simulink library "Brakes_Pedal"  (R2020a)
settings: Solver=VariableStepAuto  StartTime=0.0  StopTime=10.0  RelTol=1e-3
undefined symbols (not defined in the file): Brakes
libraries: nesl_utility x12, sdl_lib x6, fl_lib x6
Description:
  | Component of Simscape Vehicle Templates Library
  | 
  | Copyright 2018-2020 The MathWorks, Inc.
settings Model: Creator=smiller  LastModifiedBy=smiller
settings DataIOCC: ReturnWorkspaceOutputs=off
settings DebuggingCC: ArithmeticOperatorsInVariantConditions=warning
settings SFSimCC: CustomCodeUndefinedFunction=UseInterfaceOnly

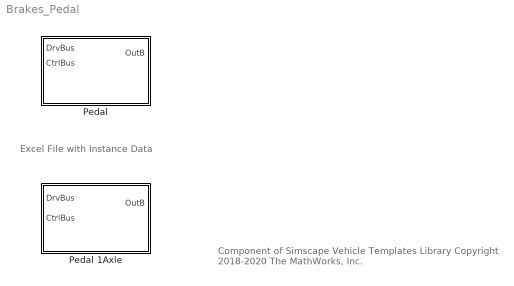
== system Brakes_Pedal ==
  note: Excel File with Instance Data
  note: Component of Simscape Vehicle Templates Library
      | Copyright 2018-2020 The MathWorks, Inc.
  Pedal : Subsystem  Tag=PublishSubsystem  VariantControl=Pedal  mask(Brake System, Pedal Input){brk_pad_rad_fa=Brakes.Front.DiscAndPad.lMeanRadius.Value, brk_pad_rad_ra=Brakes.Rear.DiscAndPad.lMeanRadius.Value, brk_cyl_bore_fa=Brakes.Front.Caliper.lCylinderDiameter.Value, brk_cyl_bore_ra=Brakes.Rear.Caliper.lCylinderDiameter.Value, brk_n_pads_fa=Brakes.Front.DiscAndPad.NPads.Value, brk_n_pads_ra=Brakes.Rear.DiscAndPad.NPads.Value, brk_mu_static_fa=Brakes.Front.DiscAndPad.rMuStatic.Value, brk_mu_static_ra=Brakes.Rear.DiscAndPad.rMuStatic.Value, brk_mu_kin_fa=Brakes.Front.DiscAndPad.rMuKinetic.Value, brk_mu_kin_ra=Brakes.Rear.DiscAndPad.rMuKinetic.Value, brk_trans_vel_fa=Brakes.Front.DiscAndPad.nTransition.Value, brk_trans_vel_ra=Brakes.Rear.DiscAndPad.nTransition.Value, brk_visc_coef_fa=Brakes.Front.DiscAndPad.dViscous.Value, brk_visc_coef_ra=Brakes.Rear.DiscAndPad.dViscous.Value, brk_max_p_fa=Brakes.Front.Caliper.pMax.Value, brk_max_p_ra=Brakes.Rear.Caliper.pMax.Value, brk_filt_fa=1/Brakes.Front.Caliper.fActuatorCutoff.Value, brk_filt_ra=1/Brakes.Rear.Caliper.fActuatorCutoff.Value}
      mask TypeOptions brk_pad_rad_fa:
      | Disc
      | Brake
      | FL/r_mean | Disc
      | Brake
      | FR/r_mean
      mask TypeOptions brk_pad_rad_ra:
      | Disc
      | Brake
      | RL/r_mean | Disc
      | Brake
      | RR/r_mean
      mask TypeOptions brk_cyl_bore_fa:
      | Disc
      | Brake
      | FL/bore | Disc
      | Brake
      | FR/bore
      mask TypeOptions brk_cyl_bore_ra:
      | Disc
      | Brake
      | RL/bore | Disc
      | Brake
      | RR/bore
      mask TypeOptions brk_n_pads_fa:
      | Disc
      | Brake
      | FL/n_pads | Disc
      | Brake
      | FR/n_pads
      mask TypeOptions brk_n_pads_ra:
      | Disc
      | Brake
      | RL/n_pads | Disc
      | Brake
      | RR/n_pads
      mask TypeOptions brk_mu_static_fa:
      | Disc
      | Brake
      | FL/mu_static | Disc
      | Brake
      | FR/mu_static
      mask TypeOptions brk_mu_static_ra:
      | Disc
      | Brake
      | RL/mu_static | Disc
      | Brake
      | RR/mu_static
      mask TypeOptions brk_mu_kin_fa:
      | Disc
      | Brake
      | FL/mu_coulomb | Disc
      | Brake
      | FR/mu_coulomb
      mask TypeOptions brk_mu_kin_ra:
      | Disc
      | Brake
      | RL/mu_coulomb | Disc
      | Brake
      | RR/mu_coulomb
      mask TypeOptions brk_trans_vel_fa:
      | Disc
      | Brake
      | FL/brkwy_vel | Disc
      | Brake
      | FR/brkwy_vel
      mask TypeOptions brk_trans_vel_ra:
      | Disc
      | Brake
      | RL/brkwy_vel | Disc
      | Brake
      | RR/brkwy_vel
      mask TypeOptions brk_visc_coef_fa:
      | Disc
      | Brake
      | FL/visc_coef | Disc
      | Brake
      | FR/visc_coef
      mask TypeOptions brk_visc_coef_ra:
      | Disc
      | Brake
      | RL/visc_coef | Disc
      | Brake
      | RR/visc_coef
      mask TypeOptions brk_max_p_fa: Actuator FL/brk_max_p | Actuator FR/brk_max_p
      mask TypeOptions brk_max_p_ra: Actuator RL/brk_max_p | Actuator RR/brk_max_p
      mask TypeOptions brk_filt_fa: Actuator FL/brk_filt | Actuator FR/brk_filt
      mask TypeOptions brk_filt_ra: Actuator RL/brk_filt | Actuator RR/brk_filt
      mask DialogControl cont_brakes Prompt: Brakes
      mask DialogControl cont_brk_geom Prompt: Geometry
      mask DialogControl text_brakes_fa Prompt: Front Susp.
      mask DialogControl text_brakes_ra Prompt: Rear Susp.
      mask DialogControl text_brakes_pad_rad Prompt: Mean Pad Radius (m)
      mask DialogControl text_brakes_cyl_bore Prompt: Cylinder Bore (m)
      mask DialogControl text_brakes_n_pads Prompt: Number of pads
      mask DialogControl cont_brk_frict Prompt: Friction
      mask DialogControl text_brakes_mu_static Prompt: Static Coeff. (0-1)
      mask DialogControl text_brakes_mu_kin Prompt: Kinetic Coeff. (0-1)
      mask DialogControl text_brakes_trans_vel Prompt: Trans. Velocity (rad/s)
      mask DialogControl text_brakes_visc_coef Prompt: Viscous (N*m/(rad/s))
      mask DialogControl cont_brk_act Prompt: Actuator
      mask DialogControl text_brakes_maxp Prompt: Max Pad Pressure (Pa)
      mask DialogControl text_brakes_filt Prompt: Time Constant (s)
      mask Display: image('sm_car_vehicle_brakes_pedal_IMAGE.png');
  Pedal 1Axle : Subsystem  Tag=PublishSubsystem  VariantControl=Pedal  mask(Brake System, Pedal Input){brk_pad_rad_fa=Brakes.Front.DiscAndPad.lMeanRadius.Value, brk_cyl_bore_fa=Brakes.Front.Caliper.lCylinderDiameter.Value, brk_n_pads_fa=Brakes.Front.DiscAndPad.NPads.Value, brk_mu_static_fa=Brakes.Front.DiscAndPad.rMuStatic.Value, brk_mu_kin_fa=Brakes.Front.DiscAndPad.rMuKinetic.Value, brk_trans_vel_fa=Brakes.Front.DiscAndPad.nTransition.Value, brk_visc_coef_fa=Brakes.Front.DiscAndPad.dViscous.Value, brk_max_p_fa=Brakes.Front.Caliper.pMax.Value, brk_filt_fa=1/Brakes.Front.Caliper.fActuatorCutoff.Value}
      mask TypeOptions brk_pad_rad_fa:
      | Disc
      | Brake
      | FL/r_mean | Disc
      | Brake
      | FR/r_mean
      mask TypeOptions brk_cyl_bore_fa:
      | Disc
      | Brake
      | FL/bore | Disc
      | Brake
      | FR/bore
      mask TypeOptions brk_n_pads_fa:
      | Disc
      | Brake
      | FL/n_pads | Disc
      | Brake
      | FR/n_pads
      mask TypeOptions brk_mu_static_fa:
      | Disc
      | Brake
      | FL/mu_static | Disc
      | Brake
      | FR/mu_static
      mask TypeOptions brk_mu_kin_fa:
      | Disc
      | Brake
      | FL/mu_coulomb | Disc
      | Brake
      | FR/mu_coulomb
      mask TypeOptions brk_trans_vel_fa:
      | Disc
      | Brake
      | FL/brkwy_vel | Disc
      | Brake
      | FR/brkwy_vel
      mask TypeOptions brk_visc_coef_fa:
      | Disc
      | Brake
      | FL/visc_coef | Disc
      | Brake
      | FR/visc_coef
      mask TypeOptions brk_max_p_fa: Actuator FL/brk_max_p | Actuator FR/brk_max_p
      mask TypeOptions brk_filt_fa: Actuator FL/brk_filt | Actuator FR/brk_filt
      mask DialogControl cont_brakes Prompt: Brakes
      mask DialogControl cont_brk_geom Prompt: Geometry
      mask DialogControl text_brakes_fa Prompt: Front Susp.
      mask DialogControl text_brakes_pad_rad Prompt: Mean Pad Radius (m)
      mask DialogControl text_brakes_cyl_bore Prompt: Cylinder Bore (m)
      mask DialogControl text_brakes_n_pads Prompt: Number of pads
      mask DialogControl cont_brk_frict Prompt: Friction
      mask DialogControl text_brakes_mu_static Prompt: Static Coeff. (0-1)
      mask DialogControl text_brakes_mu_kin Prompt: Kinetic Coeff. (0-1)
      mask DialogControl text_brakes_trans_vel Prompt: Trans. Velocity (rad/s)
      mask DialogControl text_brakes_visc_coef Prompt: Viscous (N*m/(rad/s))
      mask DialogControl cont_brk_act Prompt: Actuator
      mask DialogControl text_brakes_maxp Prompt: Max Pad Pressure (Pa)
      mask DialogControl text_brakes_filt Prompt: Time Constant (s)
      mask Display: image('sm_car_vehicle_brakes_pedal_IMAGE.png');

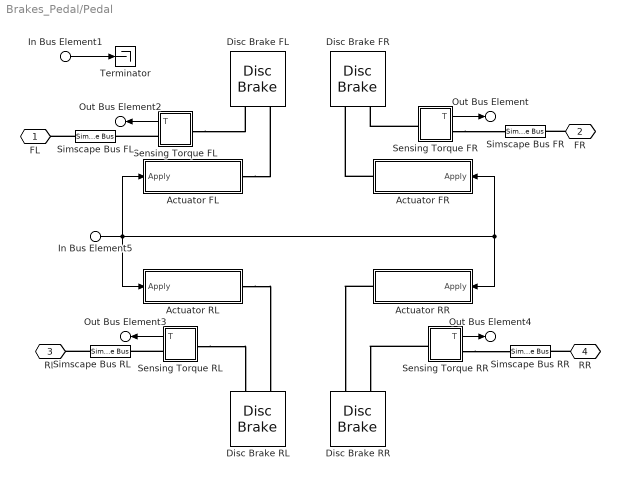
== system Brakes_Pedal/Pedal ==
  In Bus Element5 : Inport  PortName=DrvBus  Element=rBrakePedal
  In Bus Element1 : Inport  Port=2  PortName=CtrlBus
  Actuator FL : Subsystem  mask{brk_max_p=brk_max_p_fa, brk_filt=brk_filt_fa}
      mask prompts: brk_max_p "Max Pad Pressure (Pa)"; brk_filt "Time Constant (s)"
      mask TypeOptions brk_max_p: Filter/Numerator
  Actuator FR : Subsystem  mask{brk_max_p=brk_max_p_fa, brk_filt=brk_filt_fa}
      mask prompts: brk_max_p "Max Pad Pressure (Pa)"; brk_filt "Time Constant (s)"
      mask TypeOptions brk_max_p: Filter/Numerator
  Actuator RL : Subsystem  mask{brk_max_p=brk_max_p_ra, brk_filt=brk_filt_ra}
      mask prompts: brk_max_p "Max Pad Pressure (Pa)"; brk_filt "Time Constant (s)"
      mask TypeOptions brk_max_p: Filter/Numerator
  Actuator RR : Subsystem  mask{brk_max_p=brk_max_p_ra, brk_filt=brk_filt_ra}
      mask prompts: brk_max_p "Max Pad Pressure (Pa)"; brk_filt "Time Constant (s)"
      mask TypeOptions brk_max_p: Filter/Numerator
  Disc Brake FL : sdl_lib/Brakes & Detents/Rotational/Disc Brake  r_mean=brk_pad_rad_fa m  bore=brk_cyl_bore_fa m  n_pads=brk_n_pads_fa  thermal_port=simscape.enum.thermaleffects.omit  mu_static=brk_mu_static_fa  mu_coulomb=brk_mu_kin_fa  temperature_TLU=[280, 300, 320] K  mu_static_TLU=[.9, .8, .7]  mu_coulomb_TLU=[.8, .7, .6]  thermal_mass=50 kJ/K  brkwy_vel=brk_trans_vel_fa rad/s  visc_coef=brk_visc_coef_fa N*m/(rad/s)  temperature_specify=off  temperature_priority=High  temperature=300 K  temperature_nominal_specify=off  temperature_nominal_unit=K  temperature_nominal_value=1
      settings: SourceProductBaseCode=LD
  Disc Brake FR : sdl_lib/Brakes & Detents/Rotational/Disc Brake  r_mean=brk_pad_rad_fa m  bore=brk_cyl_bore_fa m  n_pads=brk_n_pads_fa  thermal_port=simscape.enum.thermaleffects.omit  mu_static=brk_mu_static_fa  mu_coulomb=brk_mu_kin_fa  temperature_TLU=[280, 300, 320] K  mu_static_TLU=[.9, .8, .7]  mu_coulomb_TLU=[.8, .7, .6]  thermal_mass=50 kJ/K  brkwy_vel=brk_trans_vel_fa rad/s  visc_coef=brk_visc_coef_fa N*m/(rad/s)  temperature_specify=off  temperature_priority=High  temperature=300 K  temperature_nominal_specify=off  temperature_nominal_unit=K  temperature_nominal_value=1
      settings: SourceProductBaseCode=LD
  Disc Brake RL : sdl_lib/Brakes & Detents/Rotational/Disc Brake  r_mean=brk_pad_rad_ra m  bore=brk_cyl_bore_ra m  n_pads=brk_n_pads_ra  thermal_port=simscape.enum.thermaleffects.omit  mu_static=brk_mu_static_ra  mu_coulomb=brk_mu_kin_ra  temperature_TLU=[280, 300, 320] K  mu_static_TLU=[.9, .8, .7]  mu_coulomb_TLU=[.8, .7, .6]  thermal_mass=50 kJ/K  brkwy_vel=brk_trans_vel_ra rad/s  visc_coef=brk_visc_coef_ra N*m/(rad/s)  temperature_specify=off  temperature_priority=High  temperature=300 K  temperature_nominal_specify=off  temperature_nominal_unit=K  temperature_nominal_value=1
      settings: SourceProductBaseCode=LD
  Disc Brake RR : sdl_lib/Brakes & Detents/Rotational/Disc Brake  r_mean=brk_pad_rad_ra m  bore=brk_cyl_bore_ra m  n_pads=brk_n_pads_ra  thermal_port=simscape.enum.thermaleffects.omit  mu_static=brk_mu_static_ra  mu_coulomb=brk_mu_kin_ra  temperature_TLU=[280, 300, 320] K  mu_static_TLU=[.9, .8, .7]  mu_coulomb_TLU=[.8, .7, .6]  thermal_mass=50 kJ/K  brkwy_vel=brk_trans_vel_ra rad/s  visc_coef=brk_visc_coef_ra N*m/(rad/s)  temperature_specify=off  temperature_priority=High  temperature=300 K  temperature_nominal_specify=off  temperature_nominal_unit=K  temperature_nominal_value=1
      settings: SourceProductBaseCode=LD
  Sensing Torque FL : Subsystem
  Sensing Torque FR : Subsystem
  Sensing Torque RL : Subsystem
  Sensing Torque RR : Subsystem
  Simscape Bus FL : SimscapeBus  HierarchyStrings=Axle1D
  Simscape Bus FR : SimscapeBus  HierarchyStrings=Axle1D
  Simscape Bus RL : SimscapeBus  HierarchyStrings=Axle1D
  Simscape Bus RR : SimscapeBus  HierarchyStrings=Axle1D
  Terminator : Terminator
  FL : PMIOPort  Side=Left
  FR : PMIOPort  Port=2  Side=Right
  RL : PMIOPort  Port=3  Side=Left
  RR : PMIOPort  Port=4  Side=Right
  Out Bus Element2 : Outport  VectorParamsAs1DForOutWhenUnconnected=off  PortName=OutB  Element=MBrakeFL
  Out Bus Element : Outport  VectorParamsAs1DForOutWhenUnconnected=off  PortName=OutB  Element=MBrakeFR
  Out Bus Element3 : Outport  VectorParamsAs1DForOutWhenUnconnected=off  PortName=OutB  Element=MBrakeRL
  Out Bus Element4 : Outport  VectorParamsAs1DForOutWhenUnconnected=off  PortName=OutB  Element=MBrakeRR
  wires:
  Sensing Torque RR/1(T) -> Out Bus Element4/1
  Sensing Torque RL/1(T) -> Out Bus Element3/1
  Sensing Torque FR/1(T) -> Out Bus Element/1
  Sensing Torque FL/1(T) -> Out Bus Element2/1
  In Bus Element1/1 -> Terminator/1
  In Bus Element5/1 -> Actuator RR/1(Apply), Actuator FR/1(Apply), Actuator FL/1(Apply), Actuator RL/1(Apply)
  connections:
  Sensing Torque RR/RConn1 -- Simscape Bus RR/LConn1
  Sensing Torque RL/RConn1 -- Simscape Bus RL/LConn1
  Sensing Torque FR/RConn1 -- Simscape Bus FR/LConn1
  Sensing Torque FL/RConn1 -- Simscape Bus FL/LConn1
  Sensing Torque FL/LConn1 -- Disc Brake FL/LConn2
  Simscape Bus FL/RConn1 -- FL/RConn1
  Sensing Torque RL/LConn1 -- Disc Brake RL/LConn2
  Simscape Bus RL/RConn1 -- RL/RConn1
  RR/RConn1 -- Simscape Bus RR/RConn1
  FR/RConn1 -- Simscape Bus FR/RConn1
  Actuator RR/RConn1 -- Disc Brake RR/LConn1
  Actuator FL/RConn1 -- Disc Brake FL/LConn1
  Actuator RL/RConn1 -- Disc Brake RL/LConn1
  Actuator FR/RConn1 -- Disc Brake FR/LConn1
  Sensing Torque FR/LConn1 -- Disc Brake FR/LConn2
  Sensing Torque RR/LConn1 -- Disc Brake RR/LConn2

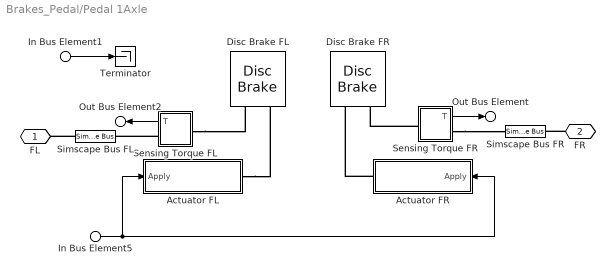
== system Brakes_Pedal/Pedal 1Axle ==
  In Bus Element5 : Inport  PortName=DrvBus  Element=rBrakePedal
  In Bus Element1 : Inport  Port=2  PortName=CtrlBus
  Actuator FL : Subsystem  mask{brk_max_p=brk_max_p_fa, brk_filt=brk_filt_fa}
      mask prompts: brk_max_p "Max Pad Pressure (Pa)"; brk_filt "Time Constant (s)"
      mask TypeOptions brk_max_p: Filter/Numerator
  Actuator FR : Subsystem  mask{brk_max_p=brk_max_p_fa, brk_filt=brk_filt_fa}
      mask prompts: brk_max_p "Max Pad Pressure (Pa)"; brk_filt "Time Constant (s)"
      mask TypeOptions brk_max_p: Filter/Numerator
  Disc Brake FL : sdl_lib/Brakes & Detents/Rotational/Disc Brake  r_mean=brk_pad_rad_fa m  bore=brk_cyl_bore_fa m  n_pads=brk_n_pads_fa  thermal_port=simscape.enum.thermaleffects.omit  mu_static=brk_mu_static_fa  mu_coulomb=brk_mu_kin_fa  temperature_TLU=[280, 300, 320] K  mu_static_TLU=[.9, .8, .7]  mu_coulomb_TLU=[.8, .7, .6]  thermal_mass=50 kJ/K  brkwy_vel=brk_trans_vel_fa rad/s  visc_coef=brk_visc_coef_fa N*m/(rad/s)  temperature_specify=off  temperature_priority=High  temperature=300 K  temperature_nominal_specify=off  temperature_nominal_unit=K  temperature_nominal_value=1
      settings: SourceProductBaseCode=LD
  Disc Brake FR : sdl_lib/Brakes & Detents/Rotational/Disc Brake  r_mean=brk_pad_rad_fa m  bore=brk_cyl_bore_fa m  n_pads=brk_n_pads_fa  thermal_port=simscape.enum.thermaleffects.omit  mu_static=brk_mu_static_fa  mu_coulomb=brk_mu_kin_fa  temperature_TLU=[280, 300, 320] K  mu_static_TLU=[.9, .8, .7]  mu_coulomb_TLU=[.8, .7, .6]  thermal_mass=50 kJ/K  brkwy_vel=brk_trans_vel_fa rad/s  visc_coef=brk_visc_coef_fa N*m/(rad/s)  temperature_specify=off  temperature_priority=High  temperature=300 K  temperature_nominal_specify=off  temperature_nominal_unit=K  temperature_nominal_value=1
      settings: SourceProductBaseCode=LD
  Sensing Torque FL : Subsystem
  Sensing Torque FR : Subsystem
  Simscape Bus FL : SimscapeBus  HierarchyStrings=Axle1D
  Simscape Bus FR : SimscapeBus  HierarchyStrings=Axle1D
  Terminator : Terminator
  FL : PMIOPort  Side=Left
  FR : PMIOPort  Port=2  Side=Right
  Out Bus Element2 : Outport  VectorParamsAs1DForOutWhenUnconnected=off  PortName=OutB  Element=MBrakeFL
  Out Bus Element : Outport  VectorParamsAs1DForOutWhenUnconnected=off  PortName=OutB  Element=MBrakeFR
  wires:
  In Bus Element5/1 -> Actuator FL/1(Apply), Actuator FR/1(Apply)
  In Bus Element1/1 -> Terminator/1
  Sensing Torque FL/1(T) -> Out Bus Element2/1
  Sensing Torque FR/1(T) -> Out Bus Element/1
  connections:
  Sensing Torque FR/LConn1 -- Disc Brake FR/LConn2
  Actuator FR/RConn1 -- Disc Brake FR/LConn1
  Actuator FL/RConn1 -- Disc Brake FL/LConn1
  FR/RConn1 -- Simscape Bus FR/RConn1
  Simscape Bus FL/RConn1 -- FL/RConn1
  Sensing Torque FL/LConn1 -- Disc Brake FL/LConn2
  Sensing Torque FL/RConn1 -- Simscape Bus FL/LConn1
  Sensing Torque FR/RConn1 -- Simscape Bus FR/LConn1

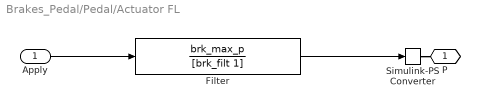
== system Brakes_Pedal/Pedal/Actuator FL ==
  Apply : Inport
  Filter : TransferFcn  Numerator=brk_max_p  Denominator=[brk_filt 1]
  Simulink-PS Converter : nesl_utility/Simulink-PS Converter  PhysicalDomain=network_engine_domain  SubClassName=ps_input  LeftPortType=input  RightPortType=output  PseudoPeriodic=off  Frequencies=[]  NoiseDistribution=none  NoiseParameters=[]  Unit=1  AffineConversion=off  FilteringAndDerivatives=provide  SimscapeFilterOrder=1  InputFilterTimeConstant=0.001  UdotUserProvided=0
  P : PMIOPort  Side=Right
  wires:
  Apply/1 -> Filter/1
  Filter/1 -> Simulink-PS Converter/1
  connections:
  Simulink-PS Converter/RConn1 -- P/RConn1

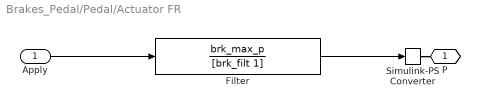
== system Brakes_Pedal/Pedal/Actuator FR ==
  Apply : Inport
  Filter : TransferFcn  Numerator=brk_max_p  Denominator=[brk_filt 1]
  Simulink-PS Converter : nesl_utility/Simulink-PS Converter  PhysicalDomain=network_engine_domain  SubClassName=ps_input  LeftPortType=input  RightPortType=output  PseudoPeriodic=off  Frequencies=[]  NoiseDistribution=none  NoiseParameters=[]  Unit=1  AffineConversion=off  FilteringAndDerivatives=provide  SimscapeFilterOrder=1  InputFilterTimeConstant=0.001  UdotUserProvided=0
  P : PMIOPort  Side=Right
  wires:
  Filter/1 -> Simulink-PS Converter/1
  Apply/1 -> Filter/1
  connections:
  Simulink-PS Converter/RConn1 -- P/RConn1

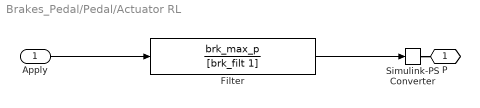
== system Brakes_Pedal/Pedal/Actuator RL ==
  Apply : Inport
  Filter : TransferFcn  Numerator=brk_max_p  Denominator=[brk_filt 1]
  Simulink-PS Converter : nesl_utility/Simulink-PS Converter  PhysicalDomain=network_engine_domain  SubClassName=ps_input  LeftPortType=input  RightPortType=output  PseudoPeriodic=off  Frequencies=[]  NoiseDistribution=none  NoiseParameters=[]  Unit=1  AffineConversion=off  FilteringAndDerivatives=provide  SimscapeFilterOrder=1  InputFilterTimeConstant=0.001  UdotUserProvided=0
  P : PMIOPort  Side=Right
  wires:
  Filter/1 -> Simulink-PS Converter/1
  Apply/1 -> Filter/1
  connections:
  Simulink-PS Converter/RConn1 -- P/RConn1

== system Brakes_Pedal/Pedal/Actuator RR ==
  Apply : Inport
  Filter : TransferFcn  Numerator=brk_max_p  Denominator=[brk_filt 1]
  Simulink-PS Converter : nesl_utility/Simulink-PS Converter  PhysicalDomain=network_engine_domain  SubClassName=ps_input  LeftPortType=input  RightPortType=output  PseudoPeriodic=off  Frequencies=[]  NoiseDistribution=none  NoiseParameters=[]  Unit=1  AffineConversion=off  FilteringAndDerivatives=provide  SimscapeFilterOrder=1  InputFilterTimeConstant=0.001  UdotUserProvided=0
  P : PMIOPort  Side=Right
  wires:
  Apply/1 -> Filter/1
  Filter/1 -> Simulink-PS Converter/1
  connections:
  Simulink-PS Converter/RConn1 -- P/RConn1

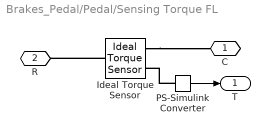
== system Brakes_Pedal/Pedal/Sensing Torque FL ==
  Ideal Torque Sensor : fl_lib/Mechanical/Mechanical Sensors/Ideal Torque Sensor
  PS-Simulink Converter : nesl_utility/PS-Simulink Converter  PhysicalDomain=network_engine_domain  SubClassName=ps_output  LeftPortType=input  RightPortType=output  PseudoPeriodic=off  Frequencies=[]  Unit=N*m  AffineConversion=off
  C : PMIOPort  Side=Right
  R : PMIOPort  Port=2  Side=Left
  T : Outport  VectorParamsAs1DForOutWhenUnconnected=off
  wires:
  PS-Simulink Converter/1 -> T/1
  connections:
  Ideal Torque Sensor/LConn1 -- R/RConn1
  Ideal Torque Sensor/RConn1 -- C/RConn1
  PS-Simulink Converter/LConn1 -- Ideal Torque Sensor/RConn2

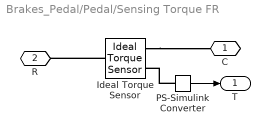
== system Brakes_Pedal/Pedal/Sensing Torque FR ==
  Ideal Torque Sensor : fl_lib/Mechanical/Mechanical Sensors/Ideal Torque Sensor
  PS-Simulink Converter : nesl_utility/PS-Simulink Converter  PhysicalDomain=network_engine_domain  SubClassName=ps_output  LeftPortType=input  RightPortType=output  PseudoPeriodic=off  Frequencies=[]  Unit=N*m  AffineConversion=off
  C : PMIOPort  Side=Right
  R : PMIOPort  Port=2  Side=Left
  T : Outport  VectorParamsAs1DForOutWhenUnconnected=off
  wires:
  PS-Simulink Converter/1 -> T/1
  connections:
  PS-Simulink Converter/LConn1 -- Ideal Torque Sensor/RConn2
  Ideal Torque Sensor/RConn1 -- C/RConn1
  Ideal Torque Sensor/LConn1 -- R/RConn1

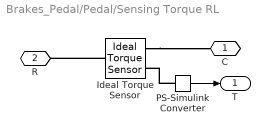
== system Brakes_Pedal/Pedal/Sensing Torque RL ==
  Ideal Torque Sensor : fl_lib/Mechanical/Mechanical Sensors/Ideal Torque Sensor
  PS-Simulink Converter : nesl_utility/PS-Simulink Converter  PhysicalDomain=network_engine_domain  SubClassName=ps_output  LeftPortType=input  RightPortType=output  PseudoPeriodic=off  Frequencies=[]  Unit=N*m  AffineConversion=off
  C : PMIOPort  Side=Right
  R : PMIOPort  Port=2  Side=Left
  T : Outport  VectorParamsAs1DForOutWhenUnconnected=off
  wires:
  PS-Simulink Converter/1 -> T/1
  connections:
  Ideal Torque Sensor/LConn1 -- R/RConn1
  Ideal Torque Sensor/RConn1 -- C/RConn1
  PS-Simulink Converter/LConn1 -- Ideal Torque Sensor/RConn2

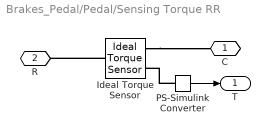
== system Brakes_Pedal/Pedal/Sensing Torque RR ==
  Ideal Torque Sensor : fl_lib/Mechanical/Mechanical Sensors/Ideal Torque Sensor
  PS-Simulink Converter : nesl_utility/PS-Simulink Converter  PhysicalDomain=network_engine_domain  SubClassName=ps_output  LeftPortType=input  RightPortType=output  PseudoPeriodic=off  Frequencies=[]  Unit=N*m  AffineConversion=off
  C : PMIOPort  Side=Right
  R : PMIOPort  Port=2  Side=Left
  T : Outport  VectorParamsAs1DForOutWhenUnconnected=off
  wires:
  PS-Simulink Converter/1 -> T/1
  connections:
  PS-Simulink Converter/LConn1 -- Ideal Torque Sensor/RConn2
  Ideal Torque Sensor/RConn1 -- C/RConn1
  Ideal Torque Sensor/LConn1 -- R/RConn1

== system Brakes_Pedal/Pedal 1Axle/Actuator FL ==
  Apply : Inport
  Filter : TransferFcn  Numerator=brk_max_p  Denominator=[brk_filt 1]
  Simulink-PS Converter : nesl_utility/Simulink-PS Converter  PhysicalDomain=network_engine_domain  SubClassName=ps_input  LeftPortType=input  RightPortType=output  PseudoPeriodic=off  Frequencies=[]  NoiseDistribution=none  NoiseParameters=[]  Unit=1  AffineConversion=off  FilteringAndDerivatives=provide  SimscapeFilterOrder=1  InputFilterTimeConstant=0.001  UdotUserProvided=0
  P : PMIOPort  Side=Right
  wires:
  Filter/1 -> Simulink-PS Converter/1
  Apply/1 -> Filter/1
  connections:
  Simulink-PS Converter/RConn1 -- P/RConn1

== system Brakes_Pedal/Pedal 1Axle/Actuator FR ==
  Apply : Inport
  Filter : TransferFcn  Numerator=brk_max_p  Denominator=[brk_filt 1]
  Simulink-PS Converter : nesl_utility/Simulink-PS Converter  PhysicalDomain=network_engine_domain  SubClassName=ps_input  LeftPortType=input  RightPortType=output  PseudoPeriodic=off  Frequencies=[]  NoiseDistribution=none  NoiseParameters=[]  Unit=1  AffineConversion=off  FilteringAndDerivatives=provide  SimscapeFilterOrder=1  InputFilterTimeConstant=0.001  UdotUserProvided=0
  P : PMIOPort  Side=Right
  wires:
  Apply/1 -> Filter/1
  Filter/1 -> Simulink-PS Converter/1
  connections:
  Simulink-PS Converter/RConn1 -- P/RConn1

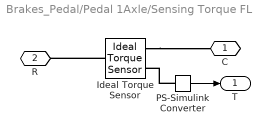
== system Brakes_Pedal/Pedal 1Axle/Sensing Torque FL ==
  Ideal Torque Sensor : fl_lib/Mechanical/Mechanical Sensors/Ideal Torque Sensor
  PS-Simulink Converter : nesl_utility/PS-Simulink Converter  PhysicalDomain=network_engine_domain  SubClassName=ps_output  LeftPortType=input  RightPortType=output  PseudoPeriodic=off  Frequencies=[]  Unit=N*m  AffineConversion=off
  C : PMIOPort  Side=Right
  R : PMIOPort  Port=2  Side=Left
  T : Outport  VectorParamsAs1DForOutWhenUnconnected=off
  wires:
  PS-Simulink Converter/1 -> T/1
  connections:
  PS-Simulink Converter/LConn1 -- Ideal Torque Sensor/RConn2
  Ideal Torque Sensor/RConn1 -- C/RConn1
  Ideal Torque Sensor/LConn1 -- R/RConn1

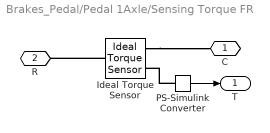
== system Brakes_Pedal/Pedal 1Axle/Sensing Torque FR ==
  Ideal Torque Sensor : fl_lib/Mechanical/Mechanical Sensors/Ideal Torque Sensor
  PS-Simulink Converter : nesl_utility/PS-Simulink Converter  PhysicalDomain=network_engine_domain  SubClassName=ps_output  LeftPortType=input  RightPortType=output  PseudoPeriodic=off  Frequencies=[]  Unit=N*m  AffineConversion=off
  C : PMIOPort  Side=Right
  R : PMIOPort  Port=2  Side=Left
  T : Outport  VectorParamsAs1DForOutWhenUnconnected=off
  wires:
  PS-Simulink Converter/1 -> T/1
  connections:
  Ideal Torque Sensor/LConn1 -- R/RConn1
  Ideal Torque Sensor/RConn1 -- C/RConn1
  PS-Simulink Converter/LConn1 -- Ideal Torque Sensor/RConn2
